simulink model "Accelator_pedal_position_sensors"  (R2023a)
settings: Solver=VariableStepAuto  StartTime=0.0  StopTime=10.0  RelTol=1e-3
libraries: simulink x4
settings Model: Creator=ItShop  LastModifiedBy=ItShop
settings DataIOCC: ReturnWorkspaceOutputs=off

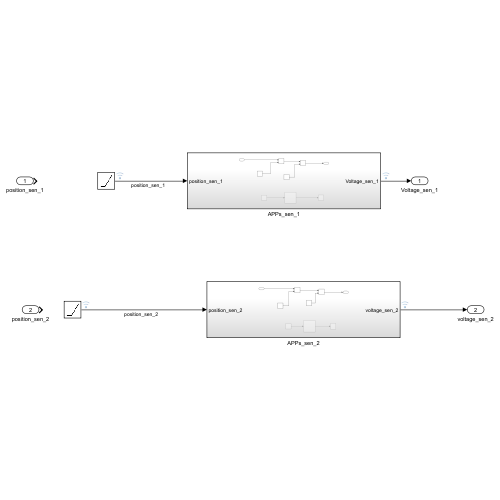
[thumbnail: Simulink's stored preview of the top-level diagram]
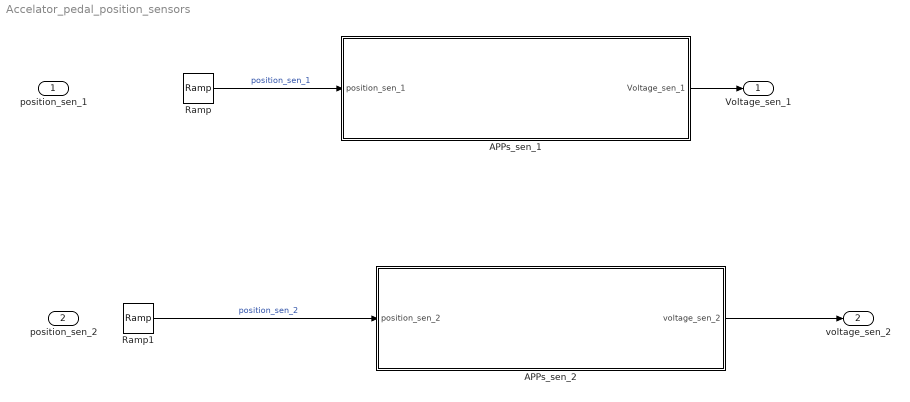
== system Accelator_pedal_position_sensors ==
  position_sen_1 : Inport
  position_sen_2 : Inport  Port=2
  APPs_sen_1 : Subsystem
  APPs_sen_2 : Subsystem
  Ramp : simulink/Sources/Ramp  slope=4  start=0  InitialOutput=.5
  Ramp1 : simulink/Sources/Ramp  slope=-4  start=0  InitialOutput=4.5
  Voltage_sen_1 : Outport
  voltage_sen_2 : Outport  Port=2
  wires:
  Ramp/1 -> APPs_sen_1/1(position_sen_1)  "position_sen_1"
  APPs_sen_1/1(Voltage_sen_1) -> Voltage_sen_1/1
  APPs_sen_2/1(voltage_sen_2) -> voltage_sen_2/1
  Ramp1/1 -> APPs_sen_2/1(position_sen_2)  "position_sen_2"

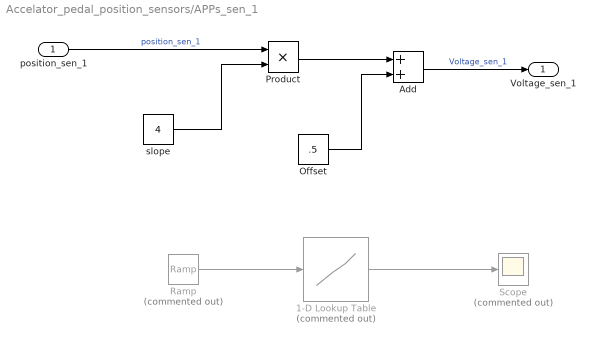
== system Accelator_pedal_position_sensors/APPs_sen_1 ==
  position_sen_1 : Inport
  1-D Lookup Table : Lookup_n-D  Commented=on  NumberOfTableDimensions=1  BreakpointsForDimension1=[0 .5 1]  Table=[.5 2.5 4.5]  InternalRulePriority=Speed  RndMeth=Simplest
  Add : Sum
  Offset : Constant  Value=.5
  Product : Product
  Ramp : simulink/Sources/Ramp  Commented=on  slope=1  start=0  InitialOutput=0
  Scope : Scope  Commented=on
  slope : Constant  Value=4
  Voltage_sen_1 : Outport
  wires:
  position_sen_1/1 -> Product/1  "position_sen_1"
  Product/1 -> Add/1
  Add/1 -> Voltage_sen_1/1  "Voltage_sen_1"
  slope/1 -> Product/2
  Offset/1 -> Add/2
  Ramp/1 -> 1-D Lookup Table/1
  1-D Lookup Table/1 -> Scope/1

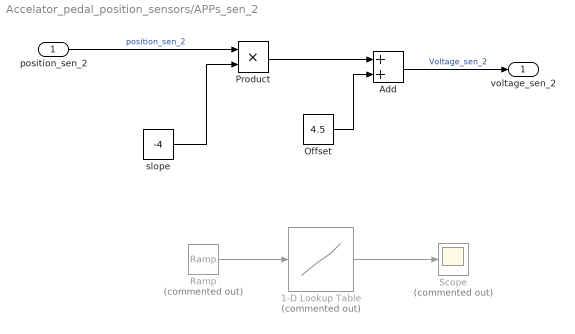
== system Accelator_pedal_position_sensors/APPs_sen_2 ==
  position_sen_2 : Inport
  1-D Lookup Table : Lookup_n-D  Commented=on  NumberOfTableDimensions=1  BreakpointsForDimension1=[0 .5 1]  Table=[4.5 2.5 .5]  InternalRulePriority=Speed  RndMeth=Simplest
  Add : Sum
  Offset : Constant  Value=4.5
  Product : Product
  Ramp : simulink/Sources/Ramp  Commented=on  slope=1  start=0  InitialOutput=0
  Scope : Scope  Commented=on
  slope : Constant  Value=-4
  voltage_sen_2 : Outport
  wires:
  position_sen_2/1 -> Product/1  "position_sen_2"
  Product/1 -> Add/1
  Offset/1 -> Add/2
  Add/1 -> voltage_sen_2/1  "Voltage_sen_2"
  slope/1 -> Product/2
  Ramp/1 -> 1-D Lookup Table/1
  1-D Lookup Table/1 -> Scope/1
